simulink model "gmsk"  (Simulink 7.9)
settings: Solver=FixedStepDiscrete  SolverMode=SingleTasking  StartTime=0.0  StopTime=1e3  RelTol=1e-3
undefined symbols (not defined in the file): EbN0, Fs, gaussfir, get, N, sided, Two
libraries: shlslibv1 x32, dspsigops x7, commutil2 x6, commsink2 x5, commdigbbndcpm2 x5, commchan3 x3, dspsnks4 x3, commrandsrc2 x1, simulink x1, dspmathops x1, commfilt2 x1, commtimrec2 x1
settings Model: synDspstartup=OK  Creator=sszilvasi  LastModifiedBy=sszilvasi
settings DataIOCC: SaveOutput=off  SignalLogging=off  SaveTime=off
settings OptimizationCC: InlineParams=on
settings DebuggingCC: AlgebraicLoopMsg=error  InheritedTsInSrcMsg=none

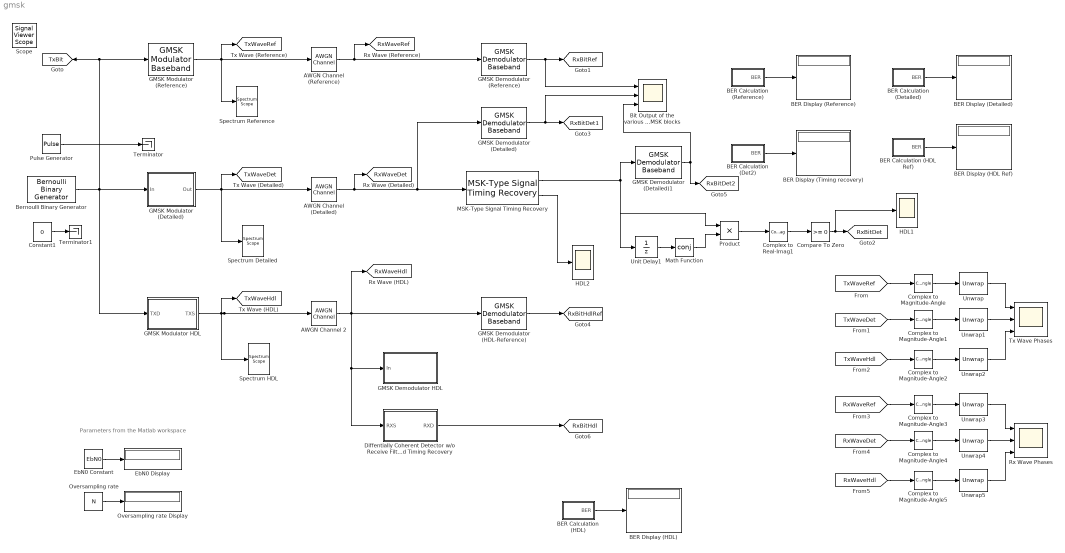
== system gmsk ==
  note: Parameters from the Matlab workspace
  AWGN Channel (Detailed) : commchan3/AWGN Channel  InputProcessing=Inherited (this choice will be removed - see release notes)  seed=67  noiseMode="Signal to noise ratio  (Eb/No)"  EbNodB=EbN0  EsNodB=10  SNRdB=10  bitsPerSym=1  Ps=1  Tsym=1  variance=1
  AWGN Channel (Reference) : commchan3/AWGN Channel  InputProcessing=Inherited (this choice will be removed - see release notes)  seed=67  noiseMode="Signal to noise ratio  (Eb/No)"  EbNodB=EbN0  EsNodB=10  SNRdB=10  bitsPerSym=1  Ps=1  Tsym=1  variance=1
  AWGN Channel 2 : commchan3/AWGN Channel  InputProcessing=Inherited (this choice will be removed - see release notes)  seed=67  noiseMode="Signal to noise ratio  (Eb/No)"  EbNodB=EbN0  EsNodB=10  SNRdB=10  bitsPerSym=1  Ps=1  Tsym=1  variance=1
  BER Calculation (Det2) : Subsystem
  BER Calculation (Detailed) : Subsystem
  BER Calculation (HDL Ref) : Subsystem
  BER Calculation (HDL) : Subsystem
  BER Calculation (Reference) : Subsystem
  BER Display (Detailed) : Display
  BER Display (HDL Ref) : Display
  BER Display (HDL) : Display
  BER Display (Reference) : Display
  BER Display (Timing recovery) : Display
  Bernoulli Binary Generator : commrandsrc2/Bernoulli Binary Generator  P=0.5  seed=61  Ts=1  frameBased=off  sampPerFrame=1  orient=off  outDataType=double
  Bit Output of the various channels demodulated with reference GMSK blocks : Scope  NumInputPorts=3
      settings: YMin=-5~-5~-5  YMax=5~5~5  SaveName=ScopeData5
  Compare To Zero : simulink/Logic and Bit Operations/Compare To Zero  relop=>=  OutDataTypeStr=boolean
  Complex to Magnitude-Angle{,1..5} (6 alike) : ComplexToMagnitudeAngle  Output=Angle
  Complex to Real-Imag1 : ComplexToRealImag  Output=Imag
  Constant1 : Constant  Value=0  SampleTime=1
  Diffentially Coherent Detector w/o Receive Filter and Timing Recovery : Subsystem
  EbN0 Constant : Constant  Value=EbN0  SampleTime=1
  EbN0 Display : Display
  GMSK Demodulator (Detailed) : commdigbbndcpm2/GMSK Demodulator Baseband  OutputType=Bit  BT=.5  pulseLength=4  preHistory=1  phaseOffset=0  samplesPerSymbol=N  RateOptions=Allow multirate processing  traceBack=16  outDType=double
  GMSK Demodulator (Detailed)1 : commdigbbndcpm2/GMSK Demodulator Baseband  OutputType=Bit  BT=.5  pulseLength=2  preHistory=1  phaseOffset=0  samplesPerSymbol=1  RateOptions=Allow multirate processing  traceBack=16  outDType=double
  GMSK Demodulator (HDL-Reference) : commdigbbndcpm2/GMSK Demodulator Baseband  OutputType=Bit  BT=.3  pulseLength=4  preHistory=1  phaseOffset=0  samplesPerSymbol=N  RateOptions=Allow multirate processing  traceBack=16  outDType=double
  GMSK Demodulator (Reference) : commdigbbndcpm2/GMSK Demodulator Baseband  OutputType=Bit  BT=.5  pulseLength=4  preHistory=1  phaseOffset=0  samplesPerSymbol=N  RateOptions=Allow multirate processing  traceBack=16  outDType=double
  GMSK Modulator (Reference) : commdigbbndcpm2/GMSK Modulator Baseband  inputType=Bit  BT=.5  pulseLength=2  preHistory=1  phaseOffset=0  samplesPerSymbol=N  RateOptions=Allow multirate processing  outDataType=double
  GMSK Demodulator HDL : Subsystem
  GMSK Modulator (Detailed) : Subsystem
  GMSK Modulator HDL : Subsystem
  HDL1 : Scope
      settings: YMin=-0.1  YMax=1.1  SaveName=ScopeData8
  HDL2 : Scope
      settings: SaveName=ScopeData3
  MSK-Type Signal Timing Recovery : commtimrec2/MSK-Type Signal Timing Recovery  modType=GMSK  sampPerSymbol=N  propGain=0.01  resetMode=None
  Math Function : Math  Operator=conj  SaturateOnIntegerOverflow=on
  Oversampling rate : Constant  Value=N  SampleTime=1
  Oversampling rate Display : Display
  Product : Product  RndMeth=Zero
  Pulse Generator : DiscretePulseGenerator  PulseType=Time based  Period=10  PulseWidth=10
  Rx Wave Phases : Scope  NumInputPorts=3
      settings: YMin=-90~-5~-5  YMax=110~5~5  SaveName=ScopeData6
  Spectrum Detailed : dspsnks4/Spectrum Scope  ScopeProperties=on  Domain=Frequency  HorizSpan=1  UseBuffer=on  BufferSize=128  Overlap=0  TreatMby1Signals=One channel  inpFftLenInherit=off  FFTlength=128  numAvg=5  DisplayProperties=off  AxisGrid=on  Memory=off  FrameNumber=on  AxisLegend=off  AxisZoom=off  OpenScopeAtSimStart=off  OpenScopeImmediately=off  FigPos=get(0,'defaultfigureposition')  AxisProperties=off  XUnits=Hertz  XRange=Two-sided ((-Fs/2...Fs/2])  XDisplay=0  InheritXIncr=on  XIncr=1.0  XLabel=Samples  XLimit=Auto  YUnits=dBW/Hertz  XMax=1  XMin=0  YLabel=Magnitude-squared, dB  LineProperties=off  wintypeSpecScope=Hann  RsSpecScope=50  betaSpecScope=5  winsampSpecScope=Periodic  XAxisParamsVer=6.9  isFrameUpgraded=on
      settings: YMin=-10  YMax=10
  Spectrum HDL : dspsnks4/Spectrum Scope  ScopeProperties=on  Domain=Frequency  HorizSpan=1  UseBuffer=on  BufferSize=128  Overlap=0  TreatMby1Signals=One channel  inpFftLenInherit=off  FFTlength=128  numAvg=5  DisplayProperties=off  AxisGrid=on  Memory=off  FrameNumber=on  AxisLegend=off  AxisZoom=off  OpenScopeAtSimStart=off  OpenScopeImmediately=off  FigPos=get(0,'defaultfigureposition')  AxisProperties=off  XUnits=Hertz  XRange=Two-sided ((-Fs/2...Fs/2])  XDisplay=0  InheritXIncr=on  XIncr=1.0  XLabel=Samples  XLimit=Auto  YUnits=dBW/Hertz  XMax=1  XMin=0  YLabel=Magnitude-squared, dB  LineProperties=off  wintypeSpecScope=Hann  RsSpecScope=50  betaSpecScope=5  winsampSpecScope=Periodic  XAxisParamsVer=6.9  isFrameUpgraded=on
      settings: YMin=-10  YMax=10
  Spectrum Reference : dspsnks4/Spectrum Scope  ScopeProperties=on  Domain=Frequency  HorizSpan=1  UseBuffer=on  BufferSize=128  Overlap=0  TreatMby1Signals=One channel  inpFftLenInherit=off  FFTlength=128  numAvg=5  DisplayProperties=off  AxisGrid=on  Memory=off  FrameNumber=on  AxisLegend=off  AxisZoom=off  OpenScopeAtSimStart=off  OpenScopeImmediately=off  FigPos=get(0,'defaultfigureposition')  AxisProperties=off  XUnits=Hertz  XRange=Two-sided ((-Fs/2...Fs/2])  XDisplay=0  InheritXIncr=on  XIncr=1.0  XLabel=Samples  XLimit=User-defined  YUnits=dBW/Hertz  XMax=8  XMin=-8  YLabel=Magnitude-squared, dB  LineProperties=off  wintypeSpecScope=Hann  RsSpecScope=50  betaSpecScope=5  winsampSpecScope=Periodic  XAxisParamsVer=6.9  isFrameUpgraded=on
      settings: YMin=-90.8889  YMax=5.0708
  Terminator : Terminator
  Terminator1 : Terminator
  Tx Wave Phases : Scope  NumInputPorts=3
      settings: YMin=-5~-5~-5  YMax=5~5~5  SaveName=ScopeData4
  Unit Delay1 : UnitDelay  SampleTime=-1
  Unwrap{,1..5} (6 alike) : dspsigops/Unwrap  tol=pi  InputProcessing=Columns as channels (frame based)  running=off
  Scope : SignalViewerScope  IOType=viewer  RefreshTime=0.035000
  tag scope: RxBitDet1=global, RxBitDet2=global, RxBitDet=global, RxBitHdl=global, RxBitHdlRef=global, RxBitRef=global, RxWaveDet=global, RxWaveHdl=global, RxWaveRef=global, TxBit=global, TxWaveDet=global, TxWaveHdl=global, TxWaveRef=global
  wires:
  MSK-Type Signal Timing Recovery/1 -> Unit Delay1/1, Product/1, GMSK Demodulator (Detailed)1/1
  Unit Delay1/1 -> Math Function/1
  Math Function/1 -> Product/2
  Product/1 -> Complex to Real-Imag1/1
  Complex to Real-Imag1/1 -> Compare To Zero/1
  GMSK Modulator (Detailed)/1(Out) -> AWGN Channel (Detailed)/1, [TxWaveDet], Spectrum Detailed/1
  AWGN Channel (Detailed)/1 -> [RxWaveDet], MSK-Type Signal Timing Recovery/1, GMSK Demodulator (Detailed)/1
  GMSK Modulator HDL/1(TXS) -> [TxWaveHdl], AWGN Channel 2/1, Spectrum HDL/1
  AWGN Channel 2/1 -> [RxWaveHdl], GMSK Demodulator (HDL-Reference)/1, GMSK Demodulator HDL/1(In), Diffentially Coherent Detector w/o Receive Filter and Timing Recovery/1(RXS)
  GMSK Modulator (Reference)/1 -> AWGN Channel (Reference)/1, [TxWaveRef], Spectrum Reference/1
  AWGN Channel (Reference)/1 -> [RxWaveRef], GMSK Demodulator (Reference)/1
  BER Calculation (Reference)/1(BER) -> BER Display (Reference)/1
  GMSK Demodulator (Reference)/1 -> [RxBitRef], Bit Output of the various channels demodulated with reference GMSK blocks/1
  Compare To Zero/1 -> [RxBitDet], HDL1/1
  GMSK Demodulator (Detailed)/1 -> [RxBitDet1], Bit Output of the various channels demodulated with reference GMSK blocks/2
  BER Calculation (Detailed)/1(BER) -> BER Display (Detailed)/1
  Bernoulli Binary Generator/1 -> [TxBit], GMSK Modulator (Reference)/1, GMSK Modulator (Detailed)/1(In), GMSK Modulator HDL/1(TXD)
  Constant1/1 -> Terminator1/1
  EbN0 Constant/1 -> EbN0 Display/1
  Oversampling rate/1 -> Oversampling rate Display/1
  MSK-Type Signal Timing Recovery/2 -> HDL2/1
  Complex to Magnitude-Angle/1 -> Unwrap/1
  Complex to Magnitude-Angle1/1 -> Unwrap1/1
  Unwrap/1 -> Tx Wave Phases/1
  Unwrap1/1 -> Tx Wave Phases/2
  [TxWaveRef] -> Complex to Magnitude-Angle/1
  [TxWaveDet] -> Complex to Magnitude-Angle1/1
  Complex to Magnitude-Angle2/1 -> Unwrap2/1
  Unwrap2/1 -> Tx Wave Phases/3
  [TxWaveHdl] -> Complex to Magnitude-Angle2/1
  Complex to Magnitude-Angle3/1 -> Unwrap3/1
  Complex to Magnitude-Angle4/1 -> Unwrap4/1
  Unwrap3/1 -> Rx Wave Phases/1
  Unwrap4/1 -> Rx Wave Phases/2
  [RxWaveRef] -> Complex to Magnitude-Angle3/1
  [RxWaveDet] -> Complex to Magnitude-Angle4/1
  Complex to Magnitude-Angle5/1 -> Unwrap5/1
  Unwrap5/1 -> Rx Wave Phases/3
  [RxWaveHdl] -> Complex to Magnitude-Angle5/1
  GMSK Demodulator (HDL-Reference)/1 -> [RxBitHdlRef]
  BER Calculation (HDL Ref)/1(BER) -> BER Display (HDL Ref)/1
  GMSK Demodulator (Detailed)1/1 -> Bit Output of the various channels demodulated with reference GMSK blocks/3, [RxBitDet2]
  BER Calculation (Det2)/1(BER) -> BER Display (Timing recovery)/1
  Pulse Generator/1 -> Terminator/1
  Diffentially Coherent Detector w/o Receive Filter and Timing Recovery/1(RXD) -> [RxBitHdl]
  BER Calculation (HDL)/1(BER) -> BER Display (HDL)/1

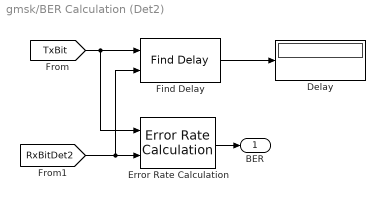
== system gmsk/BER Calculation (Det2) ==
  Delay : Display
  Error Rate Calculation : commsink2/Error Rate Calculation  N=21  st_delay=0  cp_mode=Entire frame  subframe=[]  PMode=Port  WsName=ErrorVec  RsMode2=off  stop=off  numErr=100  maxBits=1e6
  Find Delay : commutil2/Find Delay  corrLength=200  chgSigOP=off  stopUpdate=off  numConstDelay=3
  BER : Outport
  wires:
  [TxBit] -> Error Rate Calculation/1, Find Delay/1
  Error Rate Calculation/1 -> BER/1
  [RxBitDet2] -> Find Delay/2, Error Rate Calculation/2
  Find Delay/1 -> Delay/1

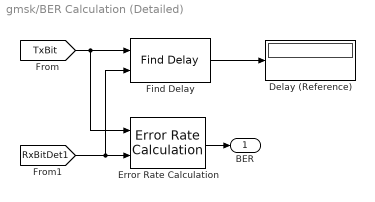
== system gmsk/BER Calculation (Detailed) ==
  Delay (Reference) : Display
  Error Rate Calculation : commsink2/Error Rate Calculation  N=16  st_delay=0  cp_mode=Entire frame  subframe=[]  PMode=Port  WsName=ErrorVec  RsMode2=off  stop=off  numErr=100  maxBits=1e6
  Find Delay : commutil2/Find Delay  corrLength=200  chgSigOP=off  stopUpdate=off  numConstDelay=3
  BER : Outport
  wires:
  [TxBit] -> Error Rate Calculation/1, Find Delay/1
  Error Rate Calculation/1 -> BER/1
  [RxBitDet1] -> Find Delay/2, Error Rate Calculation/2
  Find Delay/1 -> Delay (Reference)/1

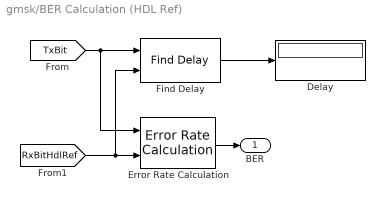
== system gmsk/BER Calculation (HDL Ref) ==
  Delay : Display
  Error Rate Calculation : commsink2/Error Rate Calculation  N=19  st_delay=0  cp_mode=Entire frame  subframe=[]  PMode=Port  WsName=ErrorVec  RsMode2=off  stop=off  numErr=100  maxBits=1e6
  Find Delay : commutil2/Find Delay  corrLength=200  chgSigOP=off  stopUpdate=off  numConstDelay=3
  BER : Outport
  wires:
  Find Delay/1 -> Delay/1
  [RxBitHdlRef] -> Error Rate Calculation/2, Find Delay/2
  Error Rate Calculation/1 -> BER/1
  [TxBit] -> Find Delay/1, Error Rate Calculation/1

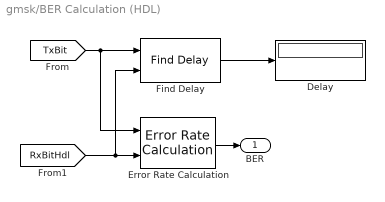
== system gmsk/BER Calculation (HDL) ==
  Delay : Display
  Error Rate Calculation : commsink2/Error Rate Calculation  N=28  st_delay=0  cp_mode=Entire frame  subframe=[]  PMode=Port  WsName=ErrorVec  RsMode2=off  stop=off  numErr=100  maxBits=1e6
  Find Delay : commutil2/Find Delay  corrLength=200  chgSigOP=off  stopUpdate=off  numConstDelay=3
  BER : Outport
  wires:
  [TxBit] -> Error Rate Calculation/1, Find Delay/1
  Error Rate Calculation/1 -> BER/1
  [RxBitHdl] -> Find Delay/2, Error Rate Calculation/2
  Find Delay/1 -> Delay/1

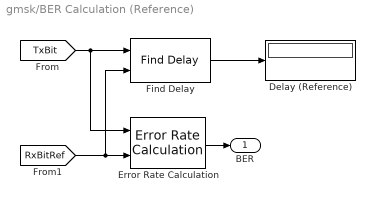
== system gmsk/BER Calculation (Reference) ==
  Delay (Reference) : Display
  Error Rate Calculation : commsink2/Error Rate Calculation  N=16  st_delay=0  cp_mode=Entire frame  subframe=[]  PMode=Port  WsName=ErrorVec  RsMode2=off  stop=off  numErr=100  maxBits=1e6
  Find Delay : commutil2/Find Delay  corrLength=200  chgSigOP=off  stopUpdate=off  numConstDelay=3
  BER : Outport
  wires:
  Find Delay/1 -> Delay (Reference)/1
  [RxBitRef] -> Error Rate Calculation/2, Find Delay/2
  Error Rate Calculation/1 -> BER/1
  [TxBit] -> Find Delay/1, Error Rate Calculation/1

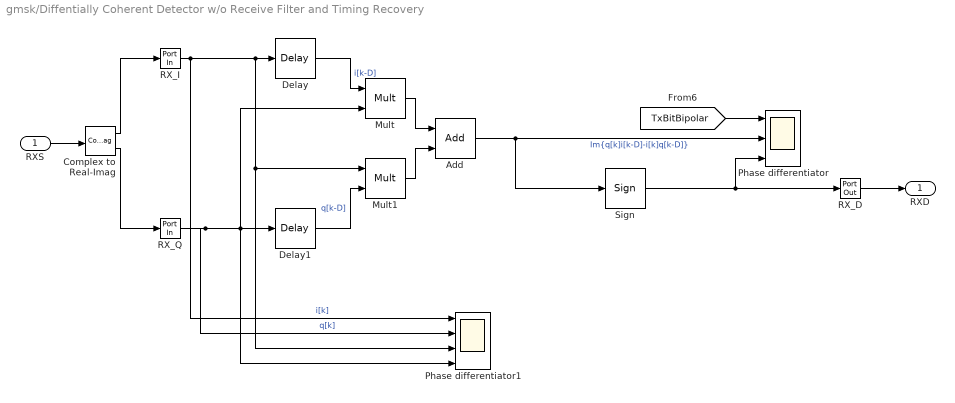
== system gmsk/Diffentially Coherent Detector w/o Receive Filter and Timing Recovery ==
  RXS : Inport
  Add : shlslibv1/Math Functions/Add  syn_add_opr=+-  syn_out_f=Full Precision  syn_out_wl=2  syn_out_fl=0  syn_out_dt=signed  syn_out_sat=off  syn_out_rnd=Floor (Truncate)  synBlockType=primitive  synLatency=0  synBlockId=96  syn_sum_of_rows=off
  Complex to Real-Imag : ComplexToRealImag
  Delay : shlslibv1/Memories/Delay  syn_delay_val=N  synBlockType=primitive  synLatency=8  synBlockId=104
  Delay1 : shlslibv1/Memories/Delay  syn_delay_val=N  synBlockType=primitive  synLatency=8  synBlockId=104
  Mult : shlslibv1/Math Functions/Mult  syn_out_f=Full Precision  syn_out_wl=16  syn_out_fl=8  syn_out_dt=signed  syn_out_sat=off  syn_out_rnd=Floor (Truncate)  synBlockType=primitive  synLatency=0  synBlockId=3  syn_opr_mode=1
  Mult1 : shlslibv1/Math Functions/Mult  syn_out_f=Full Precision  syn_out_wl=16  syn_out_fl=8  syn_out_dt=signed  syn_out_sat=off  syn_out_rnd=Floor (Truncate)  synBlockType=primitive  synLatency=0  synBlockId=3  syn_opr_mode=1
  Phase differentiator : Scope  NumInputPorts=3
      settings: YMin=-5~-5~-5  YMax=5~5~5  SaveName=ScopeData2
  Phase differentiator1 : Scope  NumInputPorts=4
      settings: YMin=-5~-5~-5~-5  YMax=5~5~5~5  SaveName=ScopeData7
  RX_D : shlslibv1/Ports & Subsystems/Port Out  syn_capture=off  syn_register=off  synBlockType=port  synLatency=0  synBlockId=1
  RX_I : shlslibv1/Ports & Subsystems/Port In  syn_out_wl=16  syn_out_fl=14  syn_out_dt=signed  syn_out_st=-1  syn_capture=off  syn_register=off  syn_out_sat=off  syn_out_rnd=off  synBlockType=port  synLatency=0  synBlockId=0
  RX_Q : shlslibv1/Ports & Subsystems/Port In  syn_out_wl=16  syn_out_fl=14  syn_out_dt=signed  syn_out_st=-1  syn_capture=off  syn_register=off  syn_out_sat=off  syn_out_rnd=off  synBlockType=port  synLatency=0  synBlockId=0
  Sign : shlslibv1/Math Functions/Sign  syn_zero_detect=on  synBlockType=custom  synLatency=0
  RXD : Outport
  wires:
  RXS/1 -> Complex to Real-Imag/1
  [TxBitBipolar] -> Phase differentiator/1
  Add/1 -> Phase differentiator/2, Sign/1  "Im{q[k]i[k-D]-i[k]q[k-D]}"
  Mult1/1 -> Add/2
  Mult/1 -> Add/1
  Delay1/1 -> Mult1/2  "q[k-D]"
  Delay/1 -> Mult/1  "i[k-D]"
  RX_I/1 -> Phase differentiator1/1, Phase differentiator1/3, Mult1/1, Delay/1  "i[k]"
  RX_Q/1 -> Phase differentiator1/2, Phase differentiator1/4, Mult/2, Delay1/1  "q[k]"
  Complex to Real-Imag/2 -> RX_Q/1
  Complex to Real-Imag/1 -> RX_I/1
  Sign/1 -> Phase differentiator/3, RX_D/1
  RX_D/1 -> RXD/1

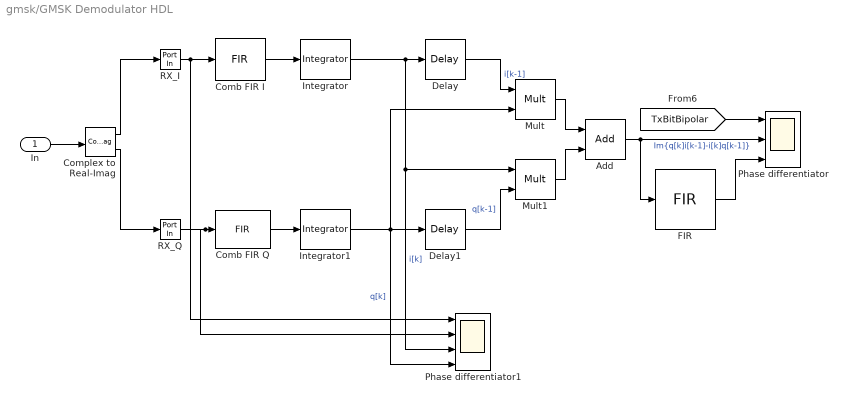
== system gmsk/GMSK Demodulator HDL ==
  In : Inport
  Add : shlslibv1/Math Functions/Add  syn_add_opr=+-  syn_out_f=Full Precision  syn_out_wl=2  syn_out_fl=0  syn_out_dt=signed  syn_out_sat=off  syn_out_rnd=Floor (Truncate)  synBlockType=primitive  synLatency=0  synBlockId=96  syn_sum_of_rows=off
  Comb FIR I : shlslibv1/Filtering/FIR  syn_coef_vec=[1 zeros(1,N-2) 1]  syn_coef_fl=8  syn_coef_rnd=Nearest  syn_show_q=off  syn_dp_f=Automatic  syn_dp_wl=16  syn_dp_fl=8  syn_dp_sat=off  syn_dp_rnd=Floor (Truncate)  syn_out_f=Full Precision  syn_out_wl=16  syn_out_fl=8  syn_out_dt=signed  syn_out_sat=off  syn_out_rnd=Floor (Truncate)  syn_rst_port=off  syn_en_port=off  synBlockType=primitive  synLatency=0  synBlockId=80
  Comb FIR Q : shlslibv1/Filtering/FIR  syn_coef_vec=[1 zeros(1,N-2) 1]  syn_coef_fl=8  syn_coef_rnd=Nearest  syn_show_q=off  syn_dp_f=Automatic  syn_dp_wl=16  syn_dp_fl=8  syn_dp_sat=off  syn_dp_rnd=Floor (Truncate)  syn_out_f=Full Precision  syn_out_wl=16  syn_out_fl=8  syn_out_dt=signed  syn_out_sat=off  syn_out_rnd=Floor (Truncate)  syn_rst_port=off  syn_en_port=off  synBlockType=primitive  synLatency=0  synBlockId=80
  Complex to Real-Imag : ComplexToRealImag
  Delay : shlslibv1/Memories/Delay  syn_delay_val=1  synBlockType=primitive  synLatency=1  synBlockId=104
  Delay1 : shlslibv1/Memories/Delay  syn_delay_val=1  synBlockType=primitive  synLatency=1  synBlockId=104
  FIR : shlslibv1/Filtering/FIR  syn_coef_vec=1/4*ones(1,4)  syn_coef_fl=8  syn_coef_rnd=Nearest  syn_show_q=off  syn_dp_f=Automatic  syn_dp_wl=16  syn_dp_fl=8  syn_dp_sat=off  syn_dp_rnd=Floor (Truncate)  syn_out_f=Full Precision  syn_out_wl=16  syn_out_fl=8  syn_out_dt=signed  syn_out_sat=off  syn_out_rnd=Floor (Truncate)  syn_rst_port=off  syn_en_port=off  synBlockType=primitive  synLatency=0  synBlockId=80
  Integrator : shlslibv1/Filtering/Integrator  syn_pole_val=1  syn_feedback_fl=8  syn_out_f=Automatic  syn_out_wl=16  syn_out_fl=8  syn_out_dt=signed  syn_out_sat=off  syn_out_rnd=off  syn_rst_port=off  syn_en_port=off  synBlockType=custom  synLatency=0
  Integrator1 : shlslibv1/Filtering/Integrator  syn_pole_val=1  syn_feedback_fl=8  syn_out_f=Automatic  syn_out_wl=16  syn_out_fl=8  syn_out_dt=signed  syn_out_sat=off  syn_out_rnd=off  syn_rst_port=off  syn_en_port=off  synBlockType=custom  synLatency=0
  Mult : shlslibv1/Math Functions/Mult  syn_out_f=Full Precision  syn_out_wl=16  syn_out_fl=8  syn_out_dt=signed  syn_out_sat=off  syn_out_rnd=Floor (Truncate)  synBlockType=primitive  synLatency=0  synBlockId=3  syn_opr_mode=1
  Mult1 : shlslibv1/Math Functions/Mult  syn_out_f=Full Precision  syn_out_wl=16  syn_out_fl=8  syn_out_dt=signed  syn_out_sat=off  syn_out_rnd=Floor (Truncate)  synBlockType=primitive  synLatency=0  synBlockId=3  syn_opr_mode=1
  Phase differentiator : Scope  NumInputPorts=3
      settings: YMin=-5~-5~-5  YMax=5~5~5  SaveName=ScopeData2
  Phase differentiator1 : Scope  NumInputPorts=4
      settings: YMin=-5~-5~-5~-5  YMax=5~5~5~5  SaveName=ScopeData7
  RX_I : shlslibv1/Ports & Subsystems/Port In  syn_out_wl=16  syn_out_fl=14  syn_out_dt=signed  syn_out_st=-1  syn_capture=off  syn_register=off  syn_out_sat=off  syn_out_rnd=off  synBlockType=port  synLatency=0  synBlockId=0
  RX_Q : shlslibv1/Ports & Subsystems/Port In  syn_out_wl=16  syn_out_fl=14  syn_out_dt=signed  syn_out_st=-1  syn_capture=off  syn_register=off  syn_out_sat=off  syn_out_rnd=off  synBlockType=port  synLatency=0  synBlockId=0
  wires:
  Complex to Real-Imag/1 -> RX_I/1
  Complex to Real-Imag/2 -> RX_Q/1
  RX_Q/1 -> Phase differentiator1/2, Comb FIR Q/1
  RX_I/1 -> Phase differentiator1/1, Comb FIR I/1
  Integrator/1 -> Delay/1, Mult1/1, Phase differentiator1/3  "i[k]"
  Integrator1/1 -> Delay1/1, Mult/2, Phase differentiator1/4  "q[k]"
  Delay/1 -> Mult/1  "i[k-1]"
  Delay1/1 -> Mult1/2  "q[k-1]"
  Mult/1 -> Add/1
  Mult1/1 -> Add/2
  Add/1 -> Phase differentiator/2, FIR/1  "Im{q[k]i[k-1]-i[k]q[k-1]}"
  Comb FIR I/1 -> Integrator/1
  Comb FIR Q/1 -> Integrator1/1
  [TxBitBipolar] -> Phase differentiator/1
  FIR/1 -> Phase differentiator/3
  In/1 -> Complex to Real-Imag/1

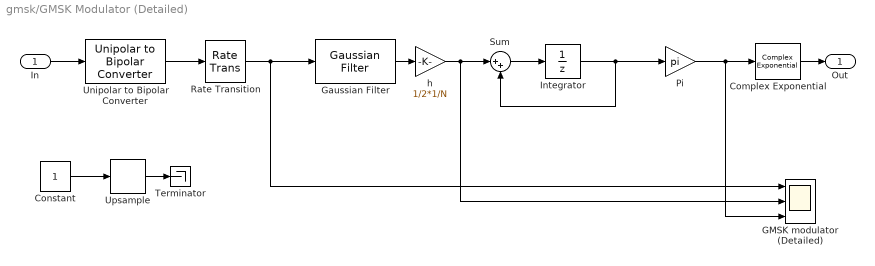
== system gmsk/GMSK Modulator (Detailed) ==
  In : Inport
  Complex Exponential : dspmathops/Complex Exponential
  Constant : Constant
  GMSK modulator (Detailed) : Scope  NumInputPorts=3
      settings: YMin=-1.5~-5~-5  YMax=1.5~5~5
  Gaussian Filter : commfilt2/Gaussian Filter  N=N  BT=.5  D=1  sampMode=Frame-based  normMode=Sum of coefficients  filterGain=1  checkCoeff=off  variableName=gaussFilt  launchFVT=off  roundingMode=Floor  overflowMode=off
  Integrator : UnitDelay  SampleTime=-1
  Pi : Gain  Gain=pi
  Rate Transition : RateTransition  OutPortSampleTime=1/N
  Sum : Sum  Inputs=|++
  Terminator : Terminator
  Unipolar to Bipolar Converter : commutil2/Unipolar to Bipolar Converter  M=2  polarity=Positive  dataType=double
  Upsample : dspsigops/Upsample  N=N  phase=0  RateOptions=Allow multirate processing  ic=1  mode=Unused parameter value
  h : Gain  Gain=1/2*1/N
  Out : Outport
  wires:
  Rate Transition/1 -> Gaussian Filter/1, GMSK modulator (Detailed)/1
  In/1 -> Unipolar to Bipolar Converter/1
  Gaussian Filter/1 -> h/1
  Complex Exponential/1 -> Out/1
  Integrator/1 -> Sum/2, Pi/1
  Sum/1 -> Integrator/1
  h/1 -> Sum/1, GMSK modulator (Detailed)/2
  Unipolar to Bipolar Converter/1 -> Rate Transition/1
  Pi/1 -> GMSK modulator (Detailed)/3, Complex Exponential/1
  Upsample/1 -> Terminator/1
  Constant/1 -> Upsample/1

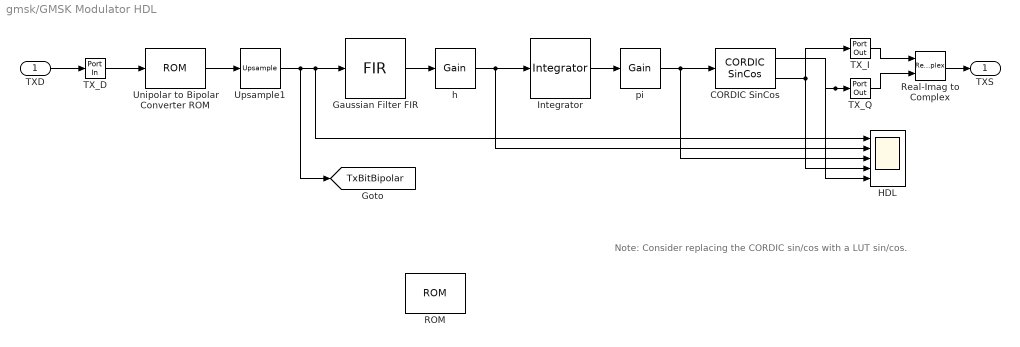
== system gmsk/GMSK Modulator HDL ==
  note: Note: Consider replacing the CORDIC sin/cos with a LUT sin/cos.
  TXD : Inport
  CORDIC SinCos : shlslibv1/CORDIC/CORDIC SinCos  syn_sincos_opr=sin&cos  syn_iter_nb=10  syn_out_wl=10  synBlockType=primitive  synLatency=12  synBlockId=53
  Gaussian Filter FIR : shlslibv1/Filtering/FIR  syn_coef_vec=gaussfir(0.5,1,N)  syn_coef_fl=15  syn_coef_rnd=Nearest  syn_show_q=off  syn_dp_f=Automatic  syn_dp_wl=16  syn_dp_fl=8  syn_dp_sat=off  syn_dp_rnd=Floor (Truncate)  syn_out_f=Full Precision  syn_out_wl=16  syn_out_fl=8  syn_out_dt=signed  syn_out_sat=off  syn_out_rnd=Floor (Truncate)  syn_rst_port=off  syn_en_port=off  synBlockType=primitive  synLatency=0  synBlockId=80
  HDL : Scope  NumInputPorts=5
      settings: YMin=-5~-5~-5~-5~-5  YMax=5~5~5~5~5
  Integrator : shlslibv1/Filtering/Integrator  syn_pole_val=1  syn_feedback_fl=8  syn_out_f=Automatic  syn_out_wl=16  syn_out_fl=8  syn_out_dt=signed  syn_out_sat=off  syn_out_rnd=off  syn_rst_port=off  syn_en_port=off  synBlockType=custom  synLatency=0
  ROM : shlslibv1/Memories/ROM  syn_rom_vec=15:-1:0  syn_out_wl=16  syn_out_fl=8  syn_out_dt=signed  syn_out_sat=off  syn_out_rnd=on  synBlockType=primitive  synLatency=1  synBlockId=62
  Real-Imag to Complex : RealImagToComplex
  TX_D : shlslibv1/Ports & Subsystems/Port In  syn_out_wl=1  syn_out_fl=0  syn_out_dt=unsigned  syn_out_st=-1  syn_capture=off  syn_register=off  syn_out_sat=off  syn_out_rnd=on  synBlockType=port  synLatency=0  synBlockId=0
  TX_I : shlslibv1/Ports & Subsystems/Port Out  syn_capture=off  syn_register=off  synBlockType=port  synLatency=0  synBlockId=1
  TX_Q : shlslibv1/Ports & Subsystems/Port Out  syn_capture=off  syn_register=off  synBlockType=port  synLatency=0  synBlockId=1
  Unipolar to Bipolar Converter ROM : shlslibv1/Memories/ROM  syn_rom_vec=[-1 1]  syn_out_wl=16  syn_out_fl=14  syn_out_dt=signed  syn_out_sat=off  syn_out_rnd=on  synBlockType=primitive  synLatency=1  synBlockId=62
  Upsample1 : shlslibv1/Signal Operations/Upsample  syn_r_val=N  syn_in_hold=on  syn_sample_offset=0  syn_sync_mode=No Sync  synBlockType=primitive  synLatency=0  synBlockId=6
  h : shlslibv1/Math Functions/Gain  syn_gain_val=1/2*1/N  syn_gain_fl=15  syn_gain_dt=signed  syn_gain_rnd=on  syn_out_f=Full Precision  syn_out_wl=16  syn_out_fl=8  syn_out_dt=signed  syn_out_sat=off  syn_out_rnd=Floor (Truncate)  synBlockType=primitive  synLatency=0  synBlockId=3  syn_opr_mode=0
  pi : shlslibv1/Math Functions/Gain  syn_gain_val=1/2  syn_gain_fl=15  syn_gain_dt=signed  syn_gain_rnd=on  syn_out_f=Full Precision  syn_out_wl=16  syn_out_fl=8  syn_out_dt=signed  syn_out_sat=off  syn_out_rnd=Floor (Truncate)  synBlockType=primitive  synLatency=0  synBlockId=3  syn_opr_mode=0
  TXS : Outport
  tag scope: TxBitBipolar=global
  wires:
  Upsample1/1 -> Gaussian Filter FIR/1, HDL/1, [TxBitBipolar]
  TX_D/1 -> Unipolar to Bipolar Converter ROM/1
  Unipolar to Bipolar Converter ROM/1 -> Upsample1/1
  Gaussian Filter FIR/1 -> h/1
  TX_I/1 -> Real-Imag to Complex/1
  TX_Q/1 -> Real-Imag to Complex/2
  h/1 -> HDL/2, Integrator/1
  Integrator/1 -> pi/1
  pi/1 -> CORDIC SinCos/1, HDL/3
  CORDIC SinCos/2 -> TX_I/1, HDL/4
  CORDIC SinCos/1 -> HDL/5, TX_Q/1
  TXD/1 -> TX_D/1
  Real-Imag to Complex/1 -> TXS/1
